simulink library "v2x_type_conv"  (R2021b)
settings: Solver=VariableStepAuto  StartTime=0.0  StopTime=10.0  RelTol=1e-3
values from neighbouring files (symbols this model uses):
  bb_ini = baseband_init()    [run_baseband_tb.m]    (also in run_v2x_baseband_tb.m = v2x_baseband_init(); run_v2x_modem_tb.m = v2x_baseband_init())
libraries: simulink x8, hdlsllib x1
settings Model: Creator=jacob  LastModifiedBy=jacob

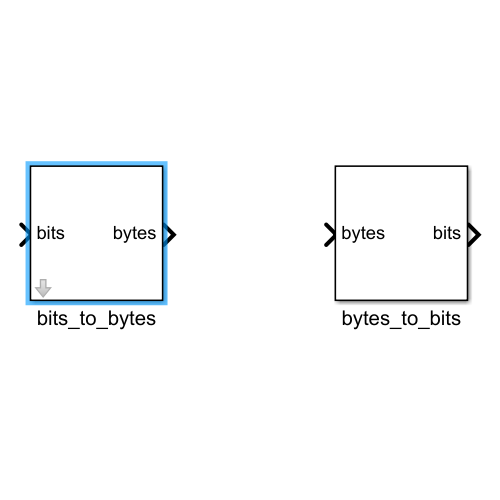
[thumbnail: Simulink's stored preview of the top-level diagram]
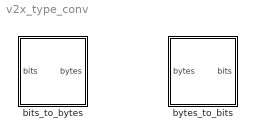
== system v2x_type_conv ==
  bits_to_bytes : Subsystem  mask{bit_frame_len=bb_ini.pkt.data_len}
      mask prompts: bit_frame_len "Bit Frame Length"
  bytes_to_bits : Subsystem

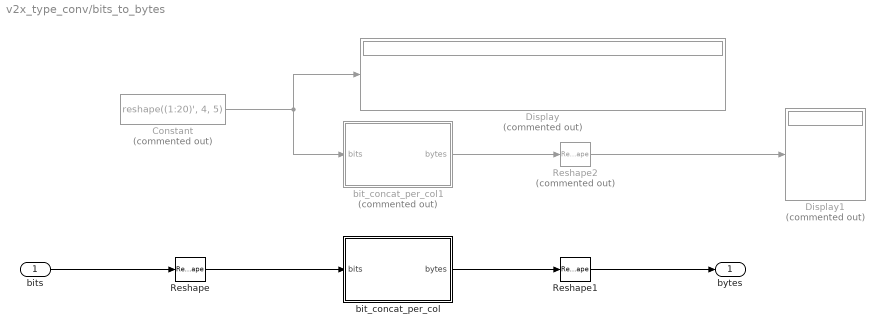
== system v2x_type_conv/bits_to_bytes ==
  bits : Inport
  Constant : Constant  Commented=on  Value=reshape((1:20)', 4, 5)  SampleTime=-1
  Display : Display  Commented=on
  Display1 : Display  Commented=on
  Reshape : Reshape  OutputDimensionality=Customize  OutputDimensions=[8, bit_frame_len/8]
  Reshape1 : Reshape  OutputDimensionality=Column vector (2-D)
  Reshape2 : Reshape  Commented=on  OutputDimensionality=Column vector (2-D)
  bit_concat_per_col : Subsystem  TreatAsAtomicUnit=on
  bit_concat_per_col1 : Subsystem  Commented=on  TreatAsAtomicUnit=on
  bytes : Outport
  wires:
  bits/1 -> Reshape/1
  bit_concat_per_col/1(bytes) -> Reshape1/1
  Reshape/1 -> bit_concat_per_col/1(bits)
  Reshape1/1 -> bytes/1
  Constant/1 -> Display/1, bit_concat_per_col1/1(bits)
  bit_concat_per_col1/1(bytes) -> Reshape2/1
  Reshape2/1 -> Display1/1

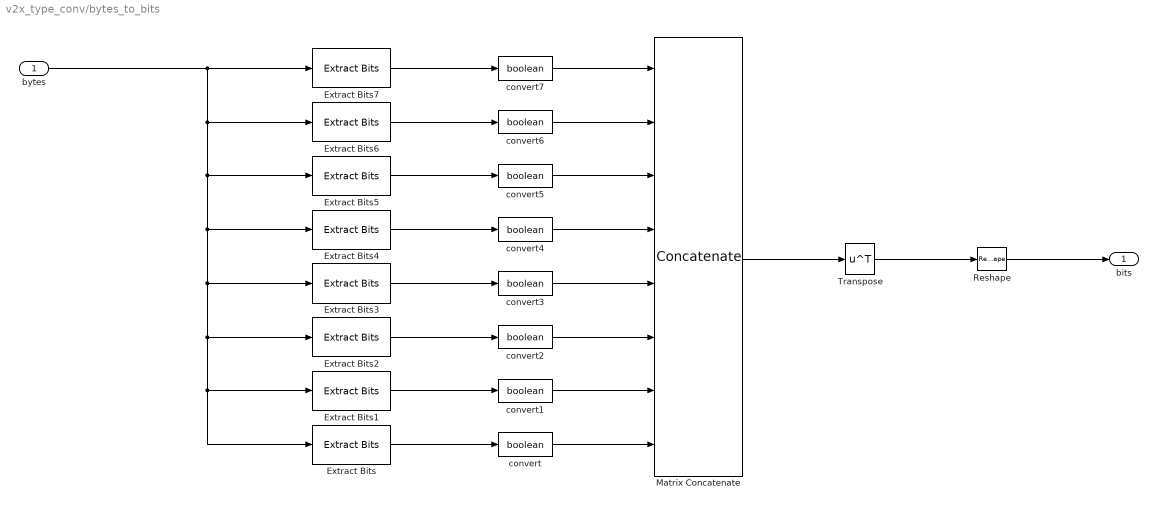
== system v2x_type_conv/bytes_to_bits ==
  bytes : Inport
  Extract Bits : simulink/Logic and Bit Operations/Extract Bits  bitsToExtract=Range of bits  numBits=8  bitIdxRange=0  outScalingMode=Treat bit field as an integer
  Extract Bits1 : simulink/Logic and Bit Operations/Extract Bits  bitsToExtract=Range of bits  numBits=8  bitIdxRange=1  outScalingMode=Treat bit field as an integer
  Extract Bits2 : simulink/Logic and Bit Operations/Extract Bits  bitsToExtract=Range of bits  numBits=8  bitIdxRange=2  outScalingMode=Treat bit field as an integer
  Extract Bits3 : simulink/Logic and Bit Operations/Extract Bits  bitsToExtract=Range of bits  numBits=8  bitIdxRange=3  outScalingMode=Treat bit field as an integer
  Extract Bits4 : simulink/Logic and Bit Operations/Extract Bits  bitsToExtract=Range of bits  numBits=8  bitIdxRange=4  outScalingMode=Treat bit field as an integer
  Extract Bits5 : simulink/Logic and Bit Operations/Extract Bits  bitsToExtract=Range of bits  numBits=8  bitIdxRange=5  outScalingMode=Treat bit field as an integer
  Extract Bits6 : simulink/Logic and Bit Operations/Extract Bits  bitsToExtract=Range of bits  numBits=8  bitIdxRange=6  outScalingMode=Treat bit field as an integer
  Extract Bits7 : simulink/Logic and Bit Operations/Extract Bits  bitsToExtract=Range of bits  numBits=8  bitIdxRange=7  outScalingMode=Treat bit field as an integer
  Matrix Concatenate : Concatenate  NumInputs=8  Mode=Multidimensional array  ConcatenateDimension=2
  Reshape : Reshape  OutputDimensionality=Column vector (2-D)
  Transpose : Math  Operator=transpose  SaturateOnIntegerOverflow=on
  convert{,1..7} (8 alike) : DataTypeConversion  OutDataTypeStr=boolean  SaturateOnIntegerOverflow=on
  bits : Outport
  wires:
  bytes/1 -> Extract Bits5/1, Extract Bits/1, Extract Bits1/1, Extract Bits2/1, Extract Bits3/1, Extract Bits4/1, Extract Bits6/1, Extract Bits7/1
  Extract Bits7/1 -> convert7/1
  Extract Bits/1 -> convert/1
  Extract Bits1/1 -> convert1/1
  Extract Bits2/1 -> convert2/1
  Extract Bits3/1 -> convert3/1
  Extract Bits4/1 -> convert4/1
  Extract Bits5/1 -> convert5/1
  Extract Bits6/1 -> convert6/1
  convert7/1 -> Matrix Concatenate/1
  convert6/1 -> Matrix Concatenate/2
  convert5/1 -> Matrix Concatenate/3
  convert4/1 -> Matrix Concatenate/4
  convert3/1 -> Matrix Concatenate/5
  convert2/1 -> Matrix Concatenate/6
  convert1/1 -> Matrix Concatenate/7
  convert/1 -> Matrix Concatenate/8
  Matrix Concatenate/1 -> Transpose/1
  Transpose/1 -> Reshape/1
  Reshape/1 -> bits/1

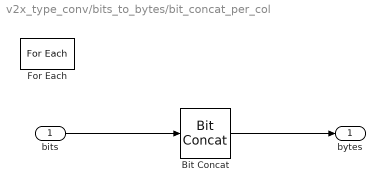
== system v2x_type_conv/bits_to_bytes/bit_concat_per_col ==
  bits : Inport  Partition=on  PartitionDimension=2  PartitionWidth=1  PartitionOffset=0
  Bit Concat : hdlsllib/Logic and Bit Operations/Bit Concat  numInputs=1
  For Each : ForEach  DisableCoverage=on
  bytes : Outport  ConcatenationDimension=1
  wires:
  bits/1 -> Bit Concat/1
  Bit Concat/1 -> bytes/1

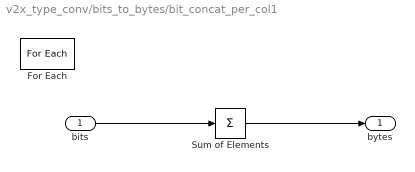
== system v2x_type_conv/bits_to_bytes/bit_concat_per_col1 ==
  bits : Inport  Partition=on  PartitionDimension=2  PartitionWidth=1  PartitionOffset=0
  For Each : ForEach  DisableCoverage=on
  Sum of Elements : Sum  Inputs=+
  bytes : Outport  ConcatenationDimension=1
  wires:
  bits/1 -> Sum of Elements/1
  Sum of Elements/1 -> bytes/1
